simulink model "trainer"  (Simulink 7.7)
settings: Solver=VariableStepDiscrete  StartTime=0.0  StopTime=10.0  RelTol=1e-3
undefined symbols (not defined in the file): serial
libraries: instrumentlib x3, simulink x1
settings Model: Creator=Jared  LastModifiedBy=Jared  SimulationMode=accelerator

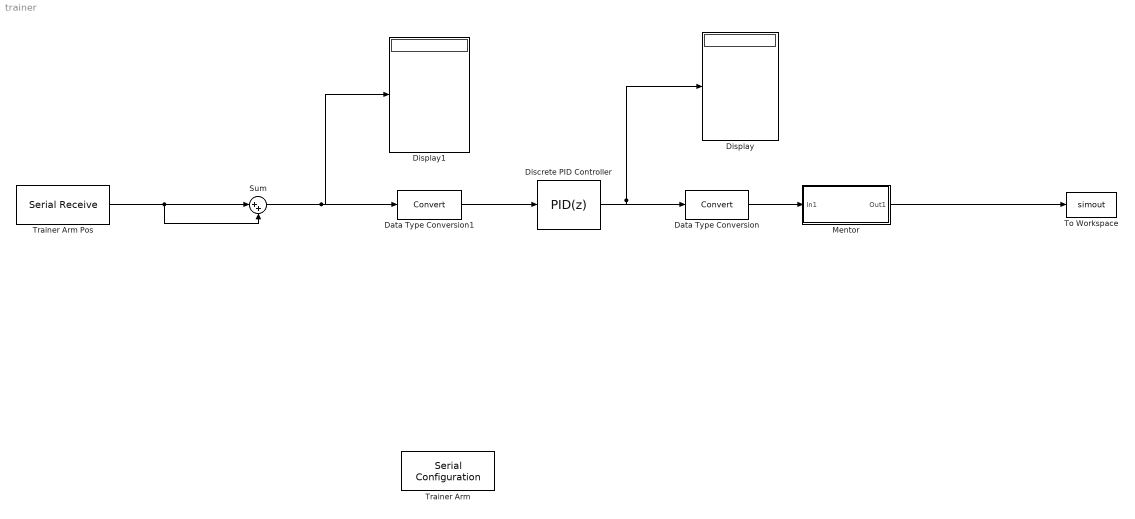
== system trainer ==
  Data Type Conversion : DataTypeConversion
  Data Type Conversion1 : DataTypeConversion
  Discrete PID Controller : simulink/Continuous/PID Controller  SystemSampleTime=-1  Controller=PID  TimeDomain=Discrete-time  SampleTime=1  IntegratorMethod=Forward Euler  FilterMethod=Forward Euler  Form=Parallel  P=1  I=1  D=0  N=100  InitialConditionSource=internal  InitialConditionForIntegrator=0  InitialConditionForFilter=0  ExternalReset=none  LimitOutput=on  UpperSaturationLimit=10000  LowerSaturationLimit=10000  LinearizeAsGain=off  AntiWindupMode=none  Kb=1  TrackingMode=off  Kt=1  PParamMin=[]  PParamMax=[]  IParamMin=[]  IParamMax=[]  DParamMin=[]  DParamMax=[]  NParamMin=[]  NParamMax=[]  KbParamMin=[]  KbParamMax=[]  KtParamMin=[]  KtParamMax=[]  POutMin=[]  POutMax=[]  IOutMin=[]  IOutMax=[]  DOutMin=[]  DOutMax=[]  NOutMin=[]  NOutMax=[]  KbOutMin=[]  KbOutMax=[]  KtOutMin=[]  KtOutMax=[]  IntegratorOutMin=[]  IntegratorOutMax=[]  FilterOutMin=[]  FilterOutMax=[]  SumOutMin=[]  SumOutMax=[]  SumI1OutMin=[]  SumI1OutMax=[]  SumI2OutMin=[]  SumI2OutMax=[]  SumI3OutMin=[]  SumI3OutMax=[]  SumDOutMin=[]  SumDOutMax=[]  SaturationOutMin=[]  SaturationOutMax=[]  IntegratorContinuousStateAttributes=''  IntegratorStateMustResolveToSignalObject=off  IntegratorRTWStateStorageClass=Auto  FilterContinuousStateAttributes=''  FilterStateMustResolveToSignalObject=off  FilterRTWStateStorageClass=Auto
  Display : Display
  Display1 : Display
  Mentor : Subsystem
  Sum : Sum  Inputs=|++
  To Workspace : ToWorkspace  VariableName=simout  SampleTime=-1  SaveFormat=Structure
  Trainer Arm : instrumentlib/Serial Configuration  Priority=-200000  ComPortMenu=COM10  ComPort=COM10  ObjConstructor=serial('COM10');  BaudRate=9600  DataBits=8  Parity=none  StopBits=1  FlowControl=none  Timeout=10  ByteOrder=LittleEndian
  Trainer Arm Pos : instrumentlib/Serial Receive  ComPortMenu=COM10  ComPort=COM10  ObjConstructor=serial('COM10');  Terminator=<none>  DataSize=6  DataType=int16  EnableBlockingMode=on  ActionDataUnavailable=Output custom value  CustomValue=-1  SampleTime=0.02
  wires:
  Discrete PID Controller/1 -> Display/1, Data Type Conversion/1
  Mentor/1(Out1) -> To Workspace/1
  Sum/1 -> Display1/1, Data Type Conversion1/1
  Trainer Arm Pos/1 -> Sum/1, Sum/2
  Data Type Conversion/1 -> Mentor/1(In1)
  Data Type Conversion1/1 -> Discrete PID Controller/1

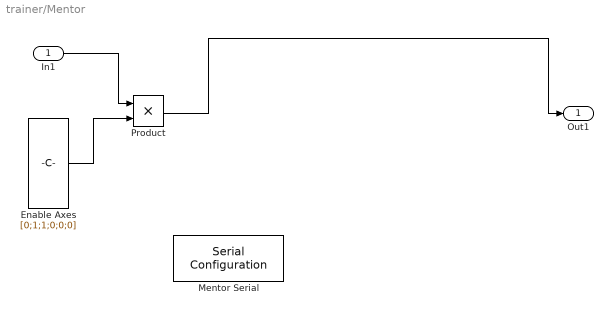
== system trainer/Mentor ==
  In1 : Inport  OutDataTypeStr=int16
  Enable Axes : Constant  Value=[0;1;1;0;0;0]
  Mentor Serial : instrumentlib/Serial Configuration  Priority=-200000  ComPortMenu=COM9  ComPort=COM9  ObjConstructor=serial('COM9');  BaudRate=9600  DataBits=8  Parity=none  StopBits=1  FlowControl=none  Timeout=10  ByteOrder=LittleEndian
  Product : Product  OutDataTypeStr=int16  RndMeth=Zero
  Out1 : Outport  OutDataTypeStr=int16
  wires:
  In1/1 -> Product/1
  Enable Axes/1 -> Product/2
  Product/1 -> Out1/1
